simulink model "Basic_Model"  (R2025a)
settings: Solver=FixedStepDiscrete  StartTime=0.0  StopTime=0.000001  FixedStep=0.000000001  RelTol=1e-3
settings Model: Creator=anunn  LastModifiedBy=anunn

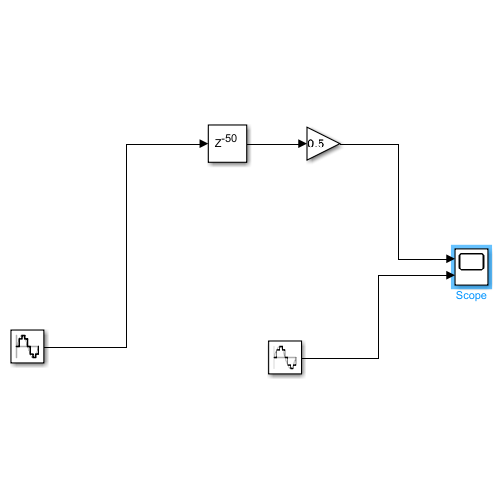
[thumbnail: Simulink's stored preview of the top-level diagram]
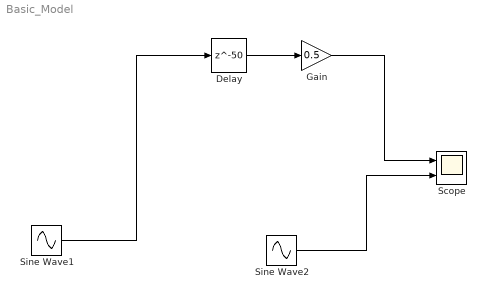
== system Basic_Model ==
  Delay : Delay  DelayLength=50
  Gain : Gain  Gain=0.5
  Scope : Scope  NumInputPorts=2
  Sine Wave1 : Sin  Frequency=628318530.71796  SampleTime=0.000000001
  Sine Wave2 : Sin  Frequency=628318530.71796  SampleTime=0.000000001
  wires:
  Sine Wave1/1 -> Delay/1
  Delay/1 -> Gain/1
  Gain/1 -> Scope/1
  Sine Wave2/1 -> Scope/2
